simulink model "main"  (R2023a)
settings: Solver=VariableStepAuto  StartTime=0.0  StopTime=5  RelTol=1e-3
libraries: spsDCVoltageSourceLib x1, spsPermanentMagnetSynchronousMachineLib x1, spsUniversalBridgeLib x1, simulink x1, spspowerguiLib x1
settings Model: Creator=13524  LastModifiedBy=13524

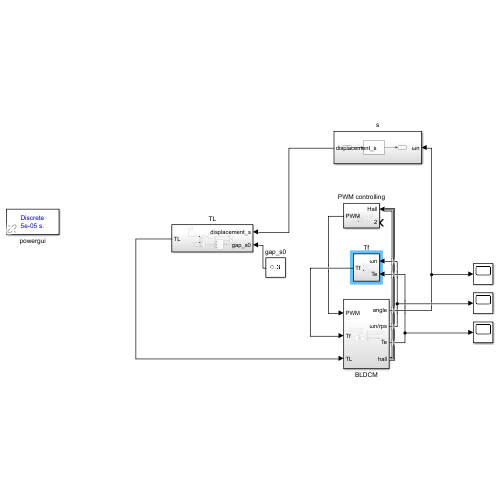
[thumbnail: Simulink's stored preview of the top-level diagram]
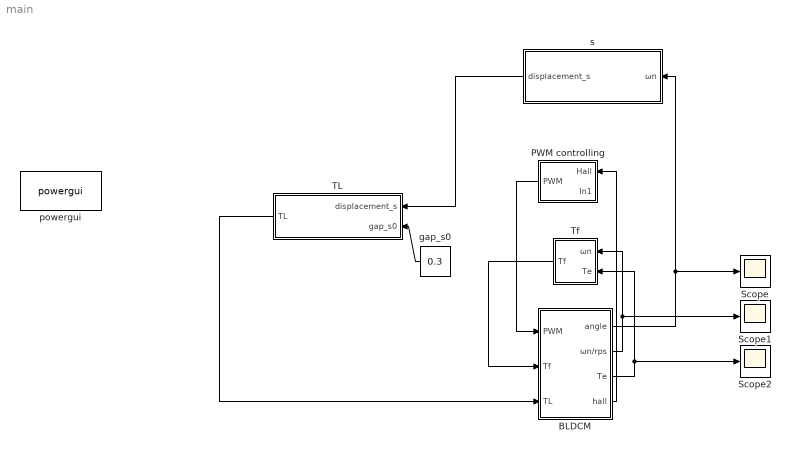
== system main ==
  BLDCM : Subsystem
  PWM controlling : Subsystem
  Scope : Scope
  Scope1 : Scope
  Scope2 : Scope
  TL : Subsystem
  Tf : Subsystem
  gap_s0 : Constant  Value=0.3  VectorParams1D=off
  powergui : spspowerguiLib/powergui  Priority=1  SimulationMode=Discrete  SampleTime=50e-6  frequency=60  Iterations=50  frequencyindice=0  Pbase=100e6  ErrMax=1e-4  UnitsV=kV  UnitsW=MW  buscounter=0  FunctionMessages=off  echomessages=off  EnableUseOfTLC=off  CurrentSourceSwitches=off  DisableSnubberDevices=off  DisableRonSwitches=off  DisableVfSwitches=off  DisplayEquations=off  AutomaticDiscreteSolvers=off  SolverType=Tustin/Backward Euler (TBE)  Interpol=off  ExternalGateDelay=off  methode=off  Ts=100  x0status=blocks  SPID=on  SwTol=0  HookPort=off  NonlinearTolerance=1e-4  nMaxIteration=100  ContinueOnMaxIteration=off  RestoreLinks=warning  ResistiveCurrentMeasurement=off  Frange=[0:2:500]  Ylog=off  Xlog=on  ShowGrid=off  save=off  variable=ZData  structure=0  ZoomFFT=off  StartTime=0.0  cycles=1  DisplayStyle=1  fundamental=60  FreqAxis=off  MaxFrequency=1000  frequencyindicesteady=1  RmsSteady=1  display=off
  s : Subsystem
  wires:
  gap_s0/1 -> TL/2(gap_s0)
  TL/1(TL) -> BLDCM/3(TL)
  s/1(displacement_s) -> TL/1(displacement_s)
  Tf/1(Tf) -> BLDCM/2(Tf)
  BLDCM/3(Te) -> Scope2/1, Tf/2(Te)
  BLDCM/2(ωn/rps) -> Scope1/1, Tf/1(ωn)
  BLDCM/1(angle) -> Scope/1, s/1(ωn)
  PWM controlling/1(PWM) -> BLDCM/1(PWM)
  BLDCM/4(hall) -> PWM controlling/1(Hall)

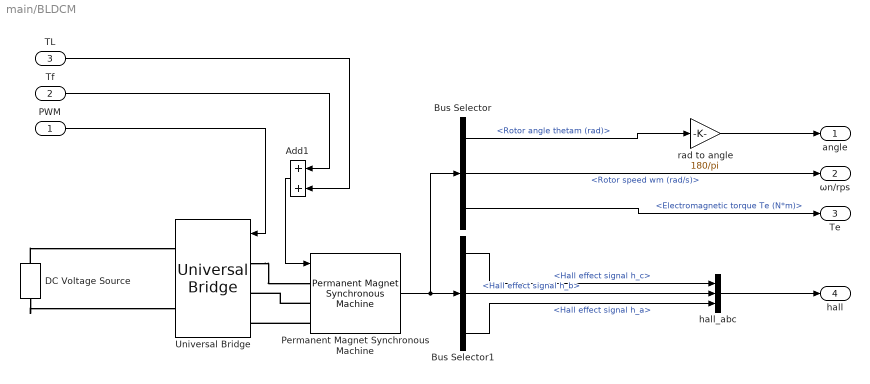
== system main/BLDCM ==
  PWM : Inport
  Tf : Inport  Port=2
  TL : Inport  Port=3
  Add1 : Sum
  Bus Selector : BusSelector  OutputSignals=Rotor angle thetam (rad),Rotor speed wm (rad/s),Electromagnetic torque Te (N*m)
  Bus Selector1 : BusSelector  OutputSignals=Hall effect signal h_c,Hall effect signal h_b,Hall effect signal h_a
  DC Voltage Source : spsDCVoltageSourceLib/DC Voltage Source  Amplitude=12  Measurements=Voltage
  Permanent Magnet Synchronous Machine : spsPermanentMagnetSynchronousMachineLib/Permanent Magnet Synchronous Machine  NbPhases=3  FluxDistribution=Trapezoidal  RotorType=Round  MechanicalLoad=Torque Tm  PresetModel=No  ShowDetailedParameters=on  MeasurementBus=off  Resistance=0.18  Inductance=0.000835  dqInductances=[8.5e-3,8.5e-3]  La=0.000395  MachineConstant=Torque Constant (N.m / A_peak)  Flux=0.19617  VoltageCst=123.2552  TorqueCst=1.177  Flat=120  Mechanical=[0.000621417 0.000303448 3]  PolePairs=4  InitialConditions=[0,0, 0,0]  InitialConditions5ph=[0 0 0 0 0 0]  RefAngle=90 degrees behind phase A axis (modified Park)  IterativeDiscreteModel=Trapezoidal non iterative  TsBlock=-1  TsPowergui=0
  Universal Bridge : spsUniversalBridgeLib/Universal Bridge  Arms=3  SnubberResistance=1e5  SnubberCapacitance=inf  Device=MOSFET / Diodes  Ron=1e-3  Lon=0  ForwardVoltages="[  0  0  ]"  ForwardVoltage=0  GTOparameters=[ 10e-6 , 20e-6 ]  IGBTparameters=[ 1e-6 , 2e-6 ]  Measurements=Device voltages  Measurements_2=None  converterType=Rectifier
  hall_abc : BusCreator  Inputs=3
  rad to angle : Gain  Gain=180/pi  OutDataTypeStr=Inherit: Same as input
  angle : Outport
  ωn/rps : Outport  Port=2
  Te : Outport  Port=3
  hall : Outport  Port=4
  wires:
  TL/1 -> Add1/2
  Bus Selector1/2 -> hall_abc/2  "<Hall effect signal h_b>"
  Add1/1 -> Permanent Magnet Synchronous Machine/1
  Bus Selector/3 -> Te/1  "<Electromagnetic torque Te (N*m)>"
  Bus Selector1/3 -> hall_abc/3  "<Hall effect signal h_a>"
  Permanent Magnet Synchronous Machine/1 -> Bus Selector/1, Bus Selector1/1
  Bus Selector1/1 -> hall_abc/1  "<Hall effect signal h_c>"
  Tf/1 -> Add1/1
  PWM/1 -> Universal Bridge/1
  Bus Selector/1 -> rad to angle/1  "<Rotor angle thetam (rad)>"
  rad to angle/1 -> angle/1
  Bus Selector/2 -> ωn/rps/1  "<Rotor speed wm (rad/s)>"
  hall_abc/1 -> hall/1
  connections:
  Permanent Magnet Synchronous Machine/LConn3 -- Universal Bridge/LConn3
  Permanent Magnet Synchronous Machine/LConn2 -- Universal Bridge/LConn2
  Universal Bridge/LConn1 -- Permanent Magnet Synchronous Machine/LConn1
  DC Voltage Source/LConn1 -- Universal Bridge/RConn2
  DC Voltage Source/RConn1 -- Universal Bridge/RConn1

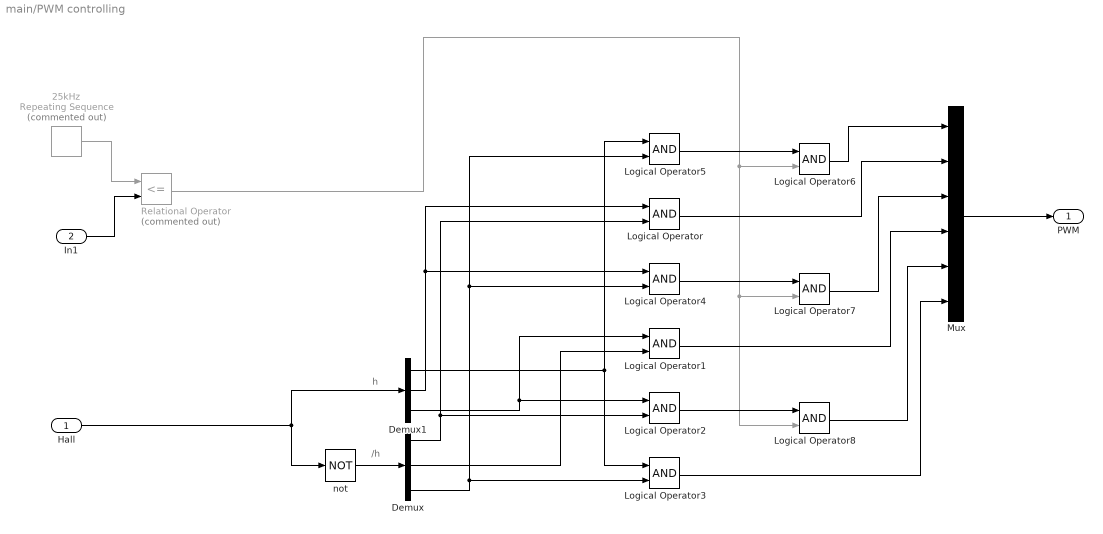
== system main/PWM controlling ==
  note: h
  note: /h
  Hall : Inport
  In1 : Inport  Port=2
  25kHz : simulink/Sources/Repeating Sequence  Commented=on  rep_seq_t="[0  1]"  rep_seq_y="[0  1]"
  Demux : Demux  Outputs=3
  Demux1 : Demux  Outputs=3
  Logical Operator{,1..8} (9 alike) : Logic  AllPortsSameDT=off  OutDataTypeStr=boolean
  Mux : Mux  Inputs=6
  Relational Operator : RelationalOperator  Commented=on  Operator=<=  OutDataTypeStr=boolean  RndMeth=Simplest  InputSameDT=off
  not : Logic  Operator=NOT  IconShape=distinctive  AllPortsSameDT=off  OutDataTypeStr=boolean
  PWM : Outport
  wires:
  Hall/1 -> not/1, Demux1/1
  Demux1/2 -> Logical Operator/1, Logical Operator4/1
  Demux/3 -> Logical Operator5/2, Logical Operator4/2, Logical Operator3/2
  Demux/1 -> Logical Operator/2, Logical Operator2/2
  Demux/2 -> Logical Operator1/2
  Logical Operator3/1 -> Mux/6
  Logical Operator7/1 -> Mux/3
  Relational Operator/1 -> Logical Operator6/2, Logical Operator7/2, Logical Operator8/2
  Mux/1 -> PWM/1
  Demux1/1 -> Logical Operator5/1, Logical Operator3/1
  Demux1/3 -> Logical Operator1/1, Logical Operator2/1
  Logical Operator5/1 -> Logical Operator6/1
  Logical Operator8/1 -> Mux/5
  Logical Operator6/1 -> Mux/1
  Logical Operator2/1 -> Logical Operator8/1
  Logical Operator/1 -> Mux/2
  Logical Operator4/1 -> Logical Operator7/1
  Logical Operator1/1 -> Mux/4
  not/1 -> Demux/1
  In1/1 -> Relational Operator/2
  25kHz/1 -> Relational Operator/1

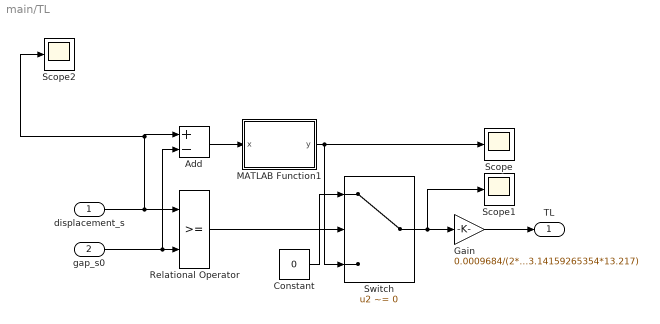
== system main/TL ==
  displacement_s : Inport
  gap_s0 : Inport  Port=2
  Add : Sum  Inputs=+-
  Constant : Constant  Value=0
  Gain : Gain  Gain=0.0009684/(2*3.14159265354*13.217)
  MATLAB Function1 : MATLAB Function  TreatAsAtomicUnit=on
  Relational Operator : RelationalOperator  OutDataTypeStr=boolean  RndMeth=Simplest  InputSameDT=off
  Scope : Scope
  Scope1 : Scope
  Scope2 : Scope
  Switch : Switch  Criteria=u2 ~= 0  ZeroCross=off  SaturateOnIntegerOverflow=off  InputSameDT=off
  TL : Outport
  wires:
  displacement_s/1 -> Scope2/1, Add/1, Relational Operator/1
  gap_s0/1 -> Add/2, Relational Operator/2
  Switch/1 -> Scope1/1, Gain/1
  Constant/1 -> Switch/1
  Add/1 -> MATLAB Function1/1(x)
  MATLAB Function1/1(y) -> Switch/3, Scope/1
  Gain/1 -> TL/1
  Relational Operator/1 -> Switch/2

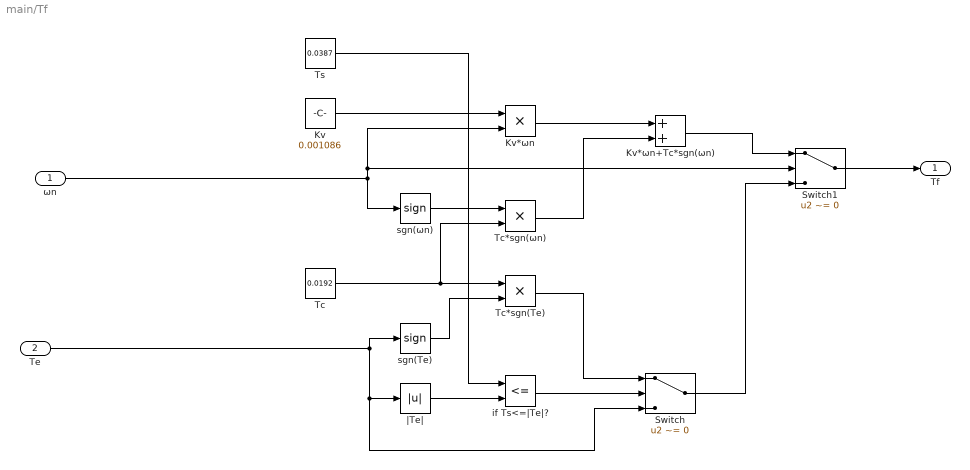
== system main/Tf ==
  ωn : Inport
  Te : Inport  Port=2
  Kv : Constant  Value=0.001086
  Kv*ωn : Product
  Kv*ωn+Tc*sgn(ωn) : Sum
  Switch : Switch  Criteria=u2 ~= 0  SaturateOnIntegerOverflow=off  InputSameDT=off
  Switch1 : Switch  Criteria=u2 ~= 0  SaturateOnIntegerOverflow=off  InputSameDT=off
  Tc : Constant  Value=0.0192
  Tc*sgn(Te) : Product
  Tc*sgn(ωn) : Product
  Ts : Constant  Value=0.0387
  if Ts<=|Te|? : RelationalOperator  Operator=<=  OutDataTypeStr=boolean  RndMeth=Simplest  InputSameDT=off
  sgn(Te) : Signum
  sgn(ωn) : Signum
  |Te| : Abs  SaturateOnIntegerOverflow=off
  Tf : Outport
  wires:
  if Ts<=|Te|?/1 -> Switch/2
  Tc/1 -> Tc*sgn(ωn)/2, Tc*sgn(Te)/1
  Ts/1 -> if Ts<=|Te|?/1
  ωn/1 -> Switch1/2, Kv*ωn/2, sgn(ωn)/1
  Kv*ωn/1 -> Kv*ωn+Tc*sgn(ωn)/1
  Tc*sgn(ωn)/1 -> Kv*ωn+Tc*sgn(ωn)/2
  Kv*ωn+Tc*sgn(ωn)/1 -> Switch1/1
  |Te|/1 -> if Ts<=|Te|?/2
  Kv/1 -> Kv*ωn/1
  Tc*sgn(Te)/1 -> Switch/1
  sgn(ωn)/1 -> Tc*sgn(ωn)/1
  sgn(Te)/1 -> Tc*sgn(Te)/2
  Te/1 -> Switch/3, |Te|/1, sgn(Te)/1
  Switch/1 -> Switch1/3
  Switch1/1 -> Tf/1

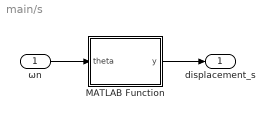
== system main/s ==
  ωn : Inport
  MATLAB Function : MATLAB Function  TreatAsAtomicUnit=on
  displacement_s : Outport
  wires:
  MATLAB Function/1(y) -> displacement_s/1
  ωn/1 -> MATLAB Function/1(theta)

== matlab function main/s/MATLAB Function ==
  data: theta input; y output
function y = fcn(theta)

y = theta.*0.9684/(2*pi*13.217);

== matlab function main/TL/MATLAB Function1 ==
  data: x input; y output
function y = fcn(x)

y=-1805*x^3+27290*x^2-6036*x+376.2;
